simulink model "test_drop_mech"  (Simulink 7.6)
settings: Solver=FixedStepDiscrete  StartTime=0.0  StopTime=0  RelTol=1e-3
undefined symbols (not defined in the file): jet, Rec, Scale_Down_B, Scale_Down_G, Scale_Down_H, Scale_Down_R, Scale_Down_S, Scale_Down_V, SDTV
libraries: vipconversions x2, vipsnks x1, vipsrcs x1, viptextngfix x1
settings Model: Creator=Thing 1  LastModifiedBy=Administrator
settings RTWCC: TargetLang=C++

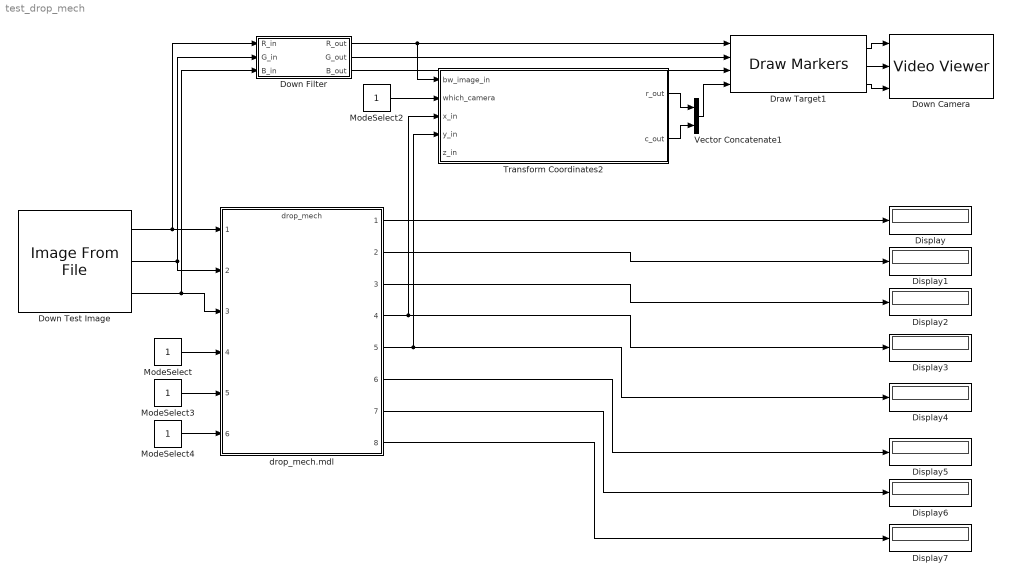
== system test_drop_mech ==
  Display{,1..7} (8 alike) : Display
  Down Camera : vipsnks/Video Viewer  DialogControllerArgs=DataTag1  inputType=Obsolete7b  imagePorts=Separate color signals  useColorMap=off  colormapValue=jet(256)  specRange=off  minInputVal=0  maxInputVal=255  FigPos=[970 679 274 199]  AxisZoom=on  trueSizedOnce=off  OpenAtMdlStart=on
  Down Filter : Subsystem
  Down Test Image : vipsrcs/Image From File  Tag=vipblks_nd  DialogController=vipDDGCreate  DialogControllerArgs=DataTag2  SystemSampleTime=-1  FileName=C:\Documents and Settings\Administrator\My Documents\Academics\Summer 2011\Newest Repository 6\src\vision\Test_Images\path9.bmp  imagePorts=Separate color signals  Ts=-1  ImageDataType=double  Signed=on  WordLength=16  sdImageDataType=uint(8)  FractionLengthMode=User-defined  FractionLength=15  OutPortLabels=R|G|B
  Draw Target1 : viptextngfix/Draw Markers  DialogController=vipDDGCreate  DialogControllerArgs=DataTag3  shape=X-mark  size=7  fill=off  fillClrSource=Specify via dialog  display=User-specified value  intensity=200  color=[0 0 0]  opacity=0.6  viewport=Entire image  antialiasing=off  inType=Obsolete  imagePorts=Separate color signals  prodOutputMode=Binary point scaling  prodOutputWordLength=32  prodOutputFracLength=14  memoryMode=Specify word length  memoryWordLength=16  memoryFracLength=15  roundingMode=Floor  overflowMode=off
  ModeSelect{,2..4} (4 alike) : Constant  SampleTime=-1
  Transform Coordinates2 : Stateflow chart  TreatAsAtomicUnit=on  SystemSampleTime=[1/30 0]
  Vector Concatenate1 : Concatenate  Mode=Multidimensional array
  drop_mech.mdl : ModelReference  ModelNameDialog=drop_mech  SimulationMode=Accelerator  ModelReferenceVersion=1.5  CopyOfModelName=drop_mech
  wires:
  Down Test Image/1 -> Down Filter/1(R_in), drop_mech.mdl/1
  Down Test Image/2 -> Down Filter/2(G_in), drop_mech.mdl/2
  Down Test Image/3 -> Down Filter/3(B_in), drop_mech.mdl/3
  Down Filter/1(R_out) -> Draw Target1/1, Transform Coordinates2/1(bw_image_in)
  Down Filter/2(G_out) -> Draw Target1/2
  Down Filter/3(B_out) -> Draw Target1/3
  ModeSelect2/1 -> Transform Coordinates2/2(which_camera)
  Transform Coordinates2/1(r_out) -> Vector Concatenate1/1
  Transform Coordinates2/2(c_out) -> Vector Concatenate1/2
  Vector Concatenate1/1 -> Draw Target1/4
  Draw Target1/1 -> Down Camera/1
  Draw Target1/2 -> Down Camera/2
  Draw Target1/3 -> Down Camera/3
  ModeSelect/1 -> drop_mech.mdl/4
  ModeSelect3/1 -> drop_mech.mdl/5
  ModeSelect4/1 -> drop_mech.mdl/6
  drop_mech.mdl/1 -> Display/1
  drop_mech.mdl/2 -> Display1/1
  drop_mech.mdl/3 -> Display2/1
  drop_mech.mdl/4 -> Display3/1, Transform Coordinates2/3(x_in)
  drop_mech.mdl/5 -> Display4/1, Transform Coordinates2/4(y_in)
  drop_mech.mdl/6 -> Display5/1
  drop_mech.mdl/7 -> Display6/1
  drop_mech.mdl/8 -> Display7/1

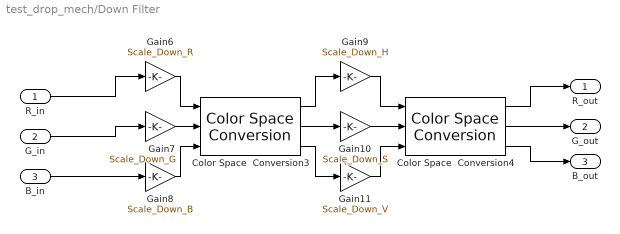
== system test_drop_mech/Down Filter ==
  R_in : Inport  PortDimensions=Down_Camera_Dimensions
  G_in : Inport  Port=2  PortDimensions=Down_Camera_Dimensions
  B_in : Inport  Port=3  PortDimensions=Down_Camera_Dimensions
  Color Space  Conversion3 : vipconversions/Color Space  Conversion  conversion=Obsolete  conversionActive=R'G'B' to HSV  wp_str=D50  rec=Rec. 601 (SDTV)  sys=1125/60/2:1  imagePorts=Separate color signals
  Color Space  Conversion4 : vipconversions/Color Space  Conversion  conversion=Obsolete  conversionActive=HSV to R'G'B'  wp_str=D50  rec=Rec. 601 (SDTV)  sys=1125/60/2:1  imagePorts=Separate color signals
  Gain10 : Gain  Gain=Scale_Down_S
  Gain11 : Gain  Gain=Scale_Down_V
  Gain6 : Gain  Gain=Scale_Down_R
  Gain7 : Gain  Gain=Scale_Down_G
  Gain8 : Gain  Gain=Scale_Down_B
  Gain9 : Gain  Gain=Scale_Down_H
  R_out : Outport  OutDataTypeStr=double
  G_out : Outport  Port=2  OutDataTypeStr=double
  B_out : Outport  Port=3  OutDataTypeStr=double
  wires:
  Gain6/1 -> Color Space  Conversion3/1
  Gain7/1 -> Color Space  Conversion3/2
  Gain8/1 -> Color Space  Conversion3/3
  Color Space  Conversion3/1 -> Gain9/1
  Color Space  Conversion3/2 -> Gain10/1
  Color Space  Conversion3/3 -> Gain11/1
  Gain9/1 -> Color Space  Conversion4/1
  Gain10/1 -> Color Space  Conversion4/2
  Gain11/1 -> Color Space  Conversion4/3
  R_in/1 -> Gain6/1
  G_in/1 -> Gain7/1
  B_in/1 -> Gain8/1
  Color Space  Conversion4/1 -> R_out/1
  Color Space  Conversion4/2 -> G_out/1
  Color Space  Conversion4/3 -> B_out/1

== matlab function Transform Coordinates2 ==
  data: bw_image_in input double; which_camera input double; x_in input double; y_in input double; r_out output double; c_out output double; z_in input double
function [r_out, c_out] = transform_G2L(bw_image_in, which_camera, x_in, y_in, z_in)
% This function, "transform Global to Local coordinates," transforms
%   global coordinates that are sent to the controller into local
%   coordinates that can be displayed over images.
%
% 5-29-11
%
% Input
%   x_in, y_in, z_in = vectors of points in global (vehicle-centered)
%     coordinate system
%   bw_image_in = a 2-D array of pixel values (used only to extract image
%     size)
%   which_camera = selects which camera for relative coordinates
%                = 0 -> Forward camera
%                = 1 -> Down camera
%
% Output
%   r_out, c_out = row, column pairs in local coordinate system

[rows, cols] = size(bw_image_in);
if( which_camera == 0 )
    r_out = z_in + floor(rows/2);
    c_out = y_in + floor(cols/2);
else
    r_out = floor(rows/2) - x_in;
    c_out = y_in + floor(cols/2);
end

return
